simulink model "fetft_dram_like_dynamic_cell"  (R2026a)
settings: Solver=ode45  StopTime=4e-05  MaxStep=5e-08
settings Model: Creator=elesamj  LastModifiedBy=elesamj

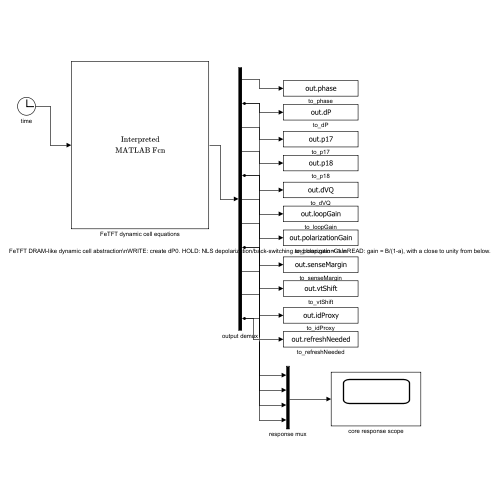
[thumbnail: Simulink's stored preview of the top-level diagram]
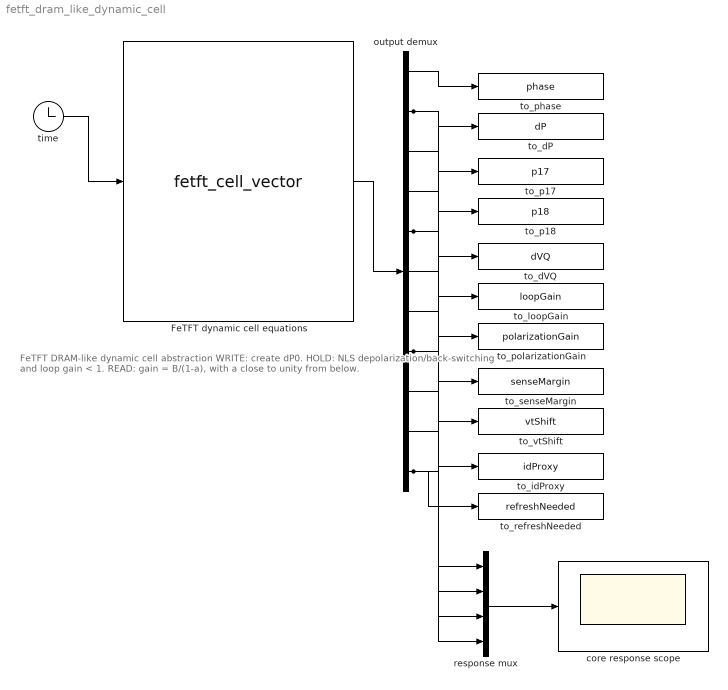
== system fetft_dram_like_dynamic_cell ==
  note: FeTFT DRAM-like dynamic cell abstraction\nWRITE: create dP0. HOLD: NLS depolarization/back-switching and loop gain < 1.\nREAD: gain = B/(1-a), with a close to unity from below.
  FeTFT dynamic cell equations : MATLABFcn  MATLABFcn=fetft_cell_vector  OutputDimensions=11
  core response scope : Scope
  output demux : Demux  Outputs=11
  response mux : Mux
  time : Clock
  to_dP : ToWorkspace  VariableName=dP  SaveFormat=Structure With Time  SampleTime=-1
  to_dVQ : ToWorkspace  VariableName=dVQ  SaveFormat=Structure With Time  SampleTime=-1
  to_idProxy : ToWorkspace  VariableName=idProxy  SaveFormat=Structure With Time  SampleTime=-1
  to_loopGain : ToWorkspace  VariableName=loopGain  SaveFormat=Structure With Time  SampleTime=-1
  to_p17 : ToWorkspace  VariableName=p17  SaveFormat=Structure With Time  SampleTime=-1
  to_p18 : ToWorkspace  VariableName=p18  SaveFormat=Structure With Time  SampleTime=-1
  to_phase : ToWorkspace  VariableName=phase  SaveFormat=Structure With Time  SampleTime=-1
  to_polarizationGain : ToWorkspace  VariableName=polarizationGain  SaveFormat=Structure With Time  SampleTime=-1
  to_refreshNeeded : ToWorkspace  VariableName=refreshNeeded  SaveFormat=Structure With Time  SampleTime=-1
  to_senseMargin : ToWorkspace  VariableName=senseMargin  SaveFormat=Structure With Time  SampleTime=-1
  to_vtShift : ToWorkspace  VariableName=vtShift  SaveFormat=Structure With Time  SampleTime=-1
  wires:
  output demux/1 -> to_phase/1
  output demux/2 -> to_dP/1, response mux/1
  output demux/3 -> to_p17/1
  output demux/4 -> to_p18/1
  output demux/5 -> to_dVQ/1, response mux/2
  output demux/6 -> to_loopGain/1
  output demux/7 -> to_polarizationGain/1
  output demux/8 -> to_senseMargin/1, response mux/3
  output demux/9 -> to_vtShift/1
  output demux/10 -> to_idProxy/1
  output demux/11 -> to_refreshNeeded/1, response mux/4
  time/1 -> FeTFT dynamic cell equations/1
  FeTFT dynamic cell equations/1 -> output demux/1
  response mux/1 -> core response scope/1
